simulink library "FloatToFixd"  (R2013b)
settings: Solver=ode45  StartTime=0.0  StopTime=10.0  RelTol=1e-3
settings Model: Creator=qzwc4r  LastModifiedBy=qzwc4r

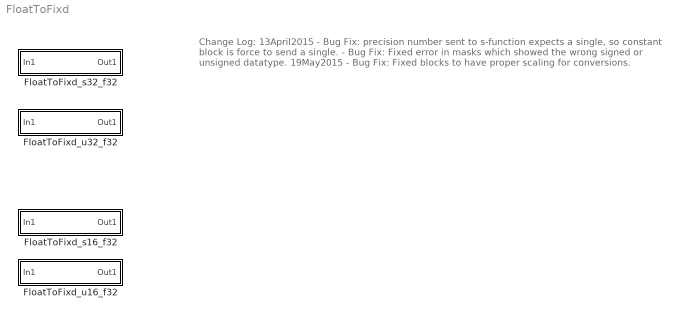
== system FloatToFixd ==
  note: Change Log:
      |
      | 13April2015
      | - Bug Fix: precision number sent to s-function expects a single, so constant block is force to send a single.
      | - Bug Fix: Fixed error in masks which showed the wrong signed or unsigned datatype.
      |
      | 19May2015
      | - Bug Fix: Fixed blocks to have proper scaling for conversions.
  FloatToFixd_s16_f32 : Subsystem  mask(FloatToFixd_s16_f32){Param1=0}
      mask prompts: Param1 "Precision"
      mask Display:
      | bits = 15;
      | pnum = Param1;
      | unum = bits-Param1;
      | 
      | port_label('input',1,'f32')
      | 
      | if pnum<0
      |     fptxt = ['s' num2str(unum) 'pm' num2str(abs(pnum))];
      |     %fprintf(['s' num2str(unum) 'pm' num2str(abs(pnum))]);
      | elseif pnum>bits
      |     fptxt = ['sm' num2str(abs(unum)) 'p' num2str(pnum)];
      |     %fprintf(['sm' num2str(abs(unum)) 'p' num2str(pnum)]);
      | else
      |     fptxt = ['s' num2str(unum) 'p' num2str(pnum)];
      |     %fprintf(['s' num2str(unum) 'p' num2str(pnum)]);
      | end
      | 
      | port_label('output',1,fptxt)
  FloatToFixd_s32_f32 : Subsystem  mask(FloatToFixd_s32_f32){Param1=0}
      mask prompts: Param1 "Precision"
      mask Display:
      | bits = 31;
      | pnum = Param1;
      | unum = bits-Param1;
      | 
      | port_label('input',1,'f32')
      | 
      | if pnum<0
      |     fptxt = ['s' num2str(unum) 'pm' num2str(abs(pnum))];
      |     %fprintf(['s' num2str(unum) 'pm' num2str(abs(pnum))]);
      | elseif pnum>bits
      |     fptxt = ['sm' num2str(abs(unum)) 'p' num2str(pnum)];
      |     %fprintf(['sm' num2str(abs(unum)) 'p' num2str(pnum)]);
      | else
      |     fptxt = ['s' num2str(unum) 'p' num2str(pnum)];
      |     %fprintf(['s' num2str(unum) 'p' num2str(pnum)]);
      | end
      | 
      | port_label('output',1,fptxt)
  FloatToFixd_u16_f32 : Subsystem  mask(FloatToFixd_u16_f32){Param1=0}
      mask prompts: Param1 "Precision"
      mask Display:
      | bits = 16;
      | pnum = Param1;
      | unum = bits-Param1;
      | 
      | port_label('input',1,'f32')
      | 
      | if pnum<0
      |     fptxt = ['u' num2str(unum) 'pm' num2str(abs(pnum))];
      | elseif pnum>bits
      |     fptxt = ['um' num2str(abs(unum)) 'p' num2str(pnum)];
      | else
      |     fptxt = ['u' num2str(unum) 'p' num2str(pnum)];
      | end
      | 
      | port_label('output',1,fptxt)
  FloatToFixd_u32_f32 : Subsystem  mask(FloatToFixd_u32_f32){Param1=0}
      mask prompts: Param1 "Precision"
      mask Display:
      | bits = 32;
      | pnum = Param1;
      | unum = bits-Param1;
      | 
      | port_label('input',1,'f32')
      | 
      | if pnum<0
      |     fptxt = ['u' num2str(unum) 'pm' num2str(abs(pnum))];
      | elseif pnum>bits
      |     fptxt = ['um' num2str(abs(unum)) 'p' num2str(pnum)];
      | else
      |     fptxt = ['u' num2str(unum) 'p' num2str(pnum)];
      | end
      | 
      | port_label('output',1,fptxt)

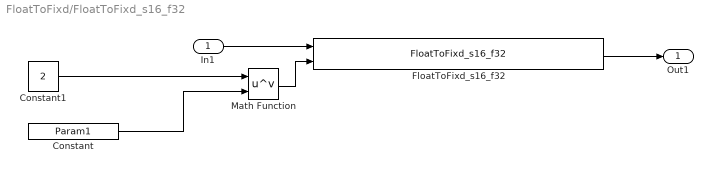
== system FloatToFixd/FloatToFixd_s16_f32 ==
  In1 : Inport
  Constant : Constant  Value=Param1  OutDataTypeStr=single
  Constant1 : Constant  Value=2  OutDataTypeStr=single
  FloatToFixd_s16_f32 : S-Function  FunctionName=FloatToFixd_s16_f32  EnableBusSupport=off  mask(Legacy Function){SFunctionSpec=int16 y1 = FloatToFixd_s16_f32(single u1, single u2), ShowSpec=on}
      mask prompts: ShowSpec "Display function specification"
      mask help:
      | This block allows you to call the legacy functions specified by the following Legacy Code Tool definition:
      | def.SFunctionName = 'FloatToFixd_s16_f32';
      | def.OutputFcnSpec = ' int16 y1 = FloatToFixd_s16_f32(single u1, single u2)';
      | def.HeaderFiles = {'NxtrFixdPt.h', 'Std_Types.h', 'Platform_Types.h', 'Compiler.h', 'Compiler_Cfg.h'};
      | def.IncPaths = {'..\SrcFiles'};
      mask Help: <p>This block was generated automatically by the Legacy Code Tool. For detailed help on this tool, call<a href="matlab:legacy_code('help')"> legacy_code('help')</a>.</p>
      mask Callback ShowSpec:
      | if strcmp(get_param(gcbh, 'ShowSpec'), 'on')
      |   set_param(gcbh, 'MaskDisplay', sprintf('fprintf(''%s'');', get_param(gcbh, 'SFunctionSpec')));
      | else
      |   set_param(gcbh, 'MaskDisplay', sprintf('fprintf(''%s'');', get_param(gcbh, 'FunctionName')));
      | end
      mask Display: fprintf('%s',' int16 y1 = FloatToFixd_s16_f32(single u1, single u2)');
  Math Function : Math  Operator=pow  SaturateOnIntegerOverflow=on
  Out1 : Outport
  wires:
  In1/1 -> FloatToFixd_s16_f32/1
  FloatToFixd_s16_f32/1 -> Out1/1
  Math Function/1 -> FloatToFixd_s16_f32/2
  Constant1/1 -> Math Function/1
  Constant/1 -> Math Function/2

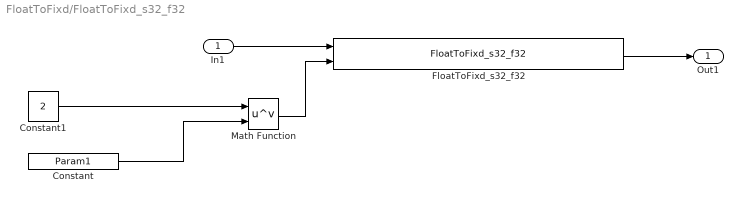
== system FloatToFixd/FloatToFixd_s32_f32 ==
  In1 : Inport
  Constant : Constant  Value=Param1  OutDataTypeStr=single
  Constant1 : Constant  Value=2  OutDataTypeStr=single
  FloatToFixd_s32_f32 : S-Function  FunctionName=FloatToFixd_s32_f32  EnableBusSupport=off  mask(Legacy Function){SFunctionSpec=int32 y1 = FloatToFixd_s32_f32(single u1, single u2), ShowSpec=on}
      mask prompts: ShowSpec "Display function specification"
      mask help:
      | This block allows you to call the legacy functions specified by the following Legacy Code Tool definition:
      | def.SFunctionName = 'FloatToFixd_s32_f32';
      | def.OutputFcnSpec = ' int32 y1 = FloatToFixd_s32_f32(single u1, single u2)';
      | def.HeaderFiles = {'NxtrFixdPt.h', 'Std_Types.h', 'Platform_Types.h', 'Compiler.h', 'Compiler_Cfg.h'};
      | def.IncPaths = {'..\SrcFiles'};
      mask Help: <p>This block was generated automatically by the Legacy Code Tool. For detailed help on this tool, call<a href="matlab:legacy_code('help')"> legacy_code('help')</a>.</p>
      mask Callback ShowSpec:
      | if strcmp(get_param(gcbh, 'ShowSpec'), 'on')
      |   set_param(gcbh, 'MaskDisplay', sprintf('fprintf(''%s'');', get_param(gcbh, 'SFunctionSpec')));
      | else
      |   set_param(gcbh, 'MaskDisplay', sprintf('fprintf(''%s'');', get_param(gcbh, 'FunctionName')));
      | end
      mask Display: fprintf(' int32 y1 = FloatToFixd_s32_f32(single u1, single u2)');
  Math Function : Math  Operator=pow  SaturateOnIntegerOverflow=on
  Out1 : Outport
  wires:
  FloatToFixd_s32_f32/1 -> Out1/1
  In1/1 -> FloatToFixd_s32_f32/1
  Constant1/1 -> Math Function/1
  Constant/1 -> Math Function/2
  Math Function/1 -> FloatToFixd_s32_f32/2

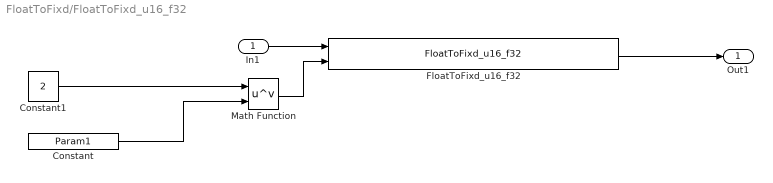
== system FloatToFixd/FloatToFixd_u16_f32 ==
  In1 : Inport
  Constant : Constant  Value=Param1  OutDataTypeStr=single
  Constant1 : Constant  Value=2  OutDataTypeStr=single
  FloatToFixd_u16_f32 : S-Function  FunctionName=FloatToFixd_u16_f32  EnableBusSupport=off  mask(Legacy Function){SFunctionSpec=uint16 y1 = FloatToFixd_u16_f32(single u1, single u2), ShowSpec=on}
      mask prompts: ShowSpec "Display function specification"
      mask help:
      | This block allows you to call the legacy functions specified by the following Legacy Code Tool definition:
      | def.SFunctionName = 'FloatToFixd_u16_f32';
      | def.OutputFcnSpec = 'uint16 y1 = FloatToFixd_u16_f32(single u1, single u2)';
      | def.HeaderFiles = {'NxtrFixdPt.h', 'Std_Types.h', 'Platform_Types.h', 'Compiler.h', 'Compiler_Cfg.h'};
      | def.IncPaths = {'..\SrcFiles'};
      mask Help: <p>This block was generated automatically by the Legacy Code Tool. For detailed help on this tool, call<a href="matlab:legacy_code('help')"> legacy_code('help')</a>.</p>
      mask Callback ShowSpec:
      | if strcmp(get_param(gcbh, 'ShowSpec'), 'on')
      |   set_param(gcbh, 'MaskDisplay', sprintf('fprintf(''%s'');', get_param(gcbh, 'SFunctionSpec')));
      | else
      |   set_param(gcbh, 'MaskDisplay', sprintf('fprintf(''%s'');', get_param(gcbh, 'FunctionName')));
      | end
      mask Display: fprintf('%s','uint16 y1 = FloatToFixd_u16_f32(single u1, single u2)');
  Math Function : Math  Operator=pow  SaturateOnIntegerOverflow=on
  Out1 : Outport
  wires:
  In1/1 -> FloatToFixd_u16_f32/1
  FloatToFixd_u16_f32/1 -> Out1/1
  Math Function/1 -> FloatToFixd_u16_f32/2
  Constant1/1 -> Math Function/1
  Constant/1 -> Math Function/2

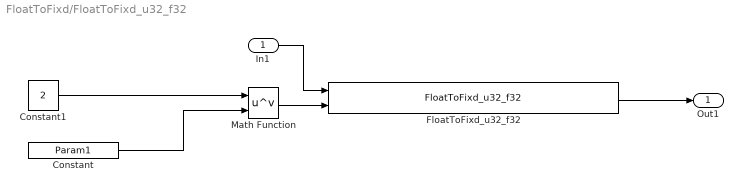
== system FloatToFixd/FloatToFixd_u32_f32 ==
  In1 : Inport
  Constant : Constant  Value=Param1  OutDataTypeStr=single
  Constant1 : Constant  Value=2  OutDataTypeStr=single
  FloatToFixd_u32_f32 : S-Function  FunctionName=FloatToFixd_u32_f32  EnableBusSupport=off  mask(Legacy Function){SFunctionSpec=uint32 y1 = FloatToFixd_u32_f32(single u1, single u2), ShowSpec=on}
      mask prompts: ShowSpec "Display function specification"
      mask help:
      | This block allows you to call the legacy functions specified by the following Legacy Code Tool definition:
      | def.SFunctionName = 'FloatToFixd_u32_f32';
      | def.OutputFcnSpec = 'uint32 y1 = FloatToFixd_u32_f32(single u1, single u2)';
      | def.HeaderFiles = {'NxtrFixdPt.h', 'Std_Types.h', 'Platform_Types.h', 'Compiler.h', 'Compiler_Cfg.h'};
      | def.IncPaths = {'..\SrcFiles'};
      mask Help: <p>This block was generated automatically by the Legacy Code Tool. For detailed help on this tool, call<a href="matlab:legacy_code('help')"> legacy_code('help')</a>.</p>
      mask Callback ShowSpec:
      | if strcmp(get_param(gcbh, 'ShowSpec'), 'on')
      |   set_param(gcbh, 'MaskDisplay', sprintf('fprintf(''%s'');', get_param(gcbh, 'SFunctionSpec')));
      | else
      |   set_param(gcbh, 'MaskDisplay', sprintf('fprintf(''%s'');', get_param(gcbh, 'FunctionName')));
      | end
      mask Display: fprintf('%s','uint32 y1 = FloatToFixd_u32_f32(single u1, single u2)');
  Math Function : Math  Operator=pow  SaturateOnIntegerOverflow=on
  Out1 : Outport
  wires:
  In1/1 -> FloatToFixd_u32_f32/1
  FloatToFixd_u32_f32/1 -> Out1/1
  Math Function/1 -> FloatToFixd_u32_f32/2
  Constant1/1 -> Math Function/1
  Constant/1 -> Math Function/2
